simulink subsystem "NoThermalEffectSSC"  (R2023b)
settings: Solver=VariableStepAuto  StartTime=0.0  StopTime=10.0  RelTol=1e-3
undefined symbols (not defined in the file): ThrmBatt, ThrmBatt1, ThrmBatt2, ThrmBatt3, ThrmBatt4, ThrmEM, ThrmEM1, ThrmEM2, ThrmEM3, ThrmEM4, ThrmPwrE
libraries: fl_lib x9
settings Model: Creator=The MathWorks, Inc.  LastModifiedBy=The MathWorks, Inc.
settings DebuggingCC: SubsystemReferenceDiagnosticForUnitTest=warning

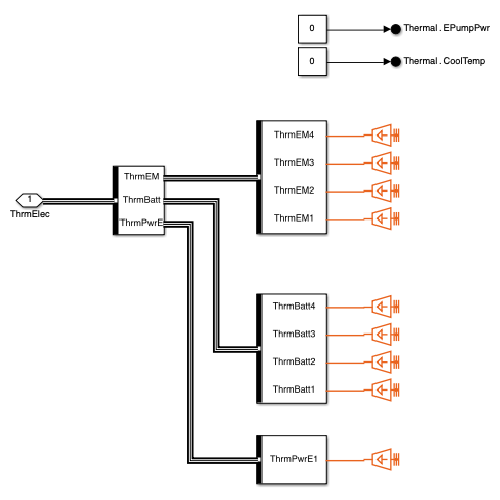
[thumbnail: Simulink's stored preview of the top-level diagram]
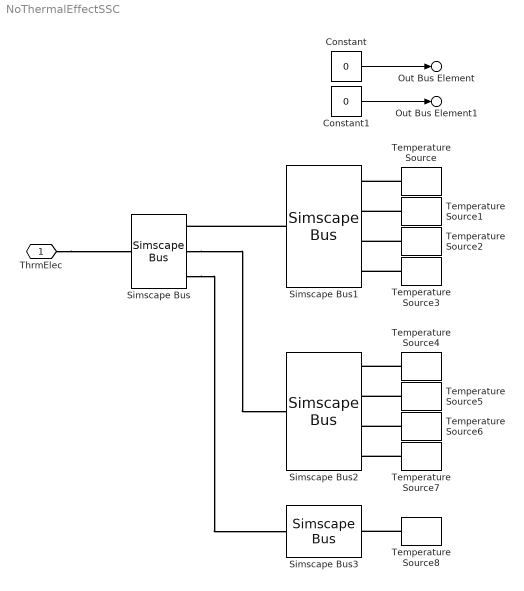
== system NoThermalEffectSSC ==
  Constant : Constant  Value=0  SampleTime=-1
  Constant1 : Constant  Value=0  SampleTime=-1
  Simscape Bus : SimscapeBus  HierarchyStrings=ThrmEM;ThrmBatt;ThrmPwrE
  Simscape Bus1 : SimscapeBus  HierarchyStrings=ThrmEM4;ThrmEM3;ThrmEM2;ThrmEM1
  Simscape Bus2 : SimscapeBus  HierarchyStrings=ThrmBatt4;ThrmBatt3;ThrmBatt2;ThrmBatt1
  Simscape Bus3 : SimscapeBus  HierarchyStrings=ThrmPwrE1
  Temperature Source{,1..3,8} (5 alike) : fl_lib/Thermal/Thermal Sources/Temperature Source  temperature=EnvAirTemp K
  Temperature Source{4..7} (4 alike) : fl_lib/Thermal/Thermal Sources/Temperature Source  temperature=PlntBattTempInitDegC degC
  ThrmElec : PMIOPort  Side=Left
  Out Bus Element : Outport  PortName=Thermal  Element=EPumpPwr
  Out Bus Element1 : Outport  PortName=Thermal  Element=CoolTemp
  wires:
  Constant1/1 -> Out Bus Element1/1
  Constant/1 -> Out Bus Element/1
  connections:
  Simscape Bus/LConn2 -- Simscape Bus2/RConn1
  Temperature Source3/LConn1 -- Simscape Bus1/LConn4
  Temperature Source5/LConn1 -- Simscape Bus2/LConn2
  Simscape Bus1/RConn1 -- Simscape Bus/LConn1
  Temperature Source4/LConn1 -- Simscape Bus2/LConn1
  Temperature Source8/LConn1 -- Simscape Bus3/LConn1
  Temperature Source6/LConn1 -- Simscape Bus2/LConn3
  Temperature Source1/LConn1 -- Simscape Bus1/LConn2
  Simscape Bus/LConn3 -- Simscape Bus3/RConn1
  Temperature Source7/LConn1 -- Simscape Bus2/LConn4
  Temperature Source2/LConn1 -- Simscape Bus1/LConn3
  Temperature Source/LConn1 -- Simscape Bus1/LConn1
  ThrmElec/RConn1 -- Simscape Bus/RConn1
